simulink model "HeliDraft_25_03_2025"  (R2024b)
settings: Solver=VariableStepAuto  StartTime=0.0  StopTime=15  RelTol=1e-3
InitFcn:
  | if exist('MTOW', 'var') == 0
  |     set_param(gcs, 'SimulationCommand', 'stop');
  |     disp('HELICOPTER PARAMETERS ARE NOT DEFINED.');
  | end
values from neighbouring files (symbols this model uses):
  R = D/2    (= 2.01773704722)    [untitled.m]
undefined symbols (not defined in the file or in its folder): AngVel, AngVeltr, BatteryCap, BatteryDischrgRate, Coeffs, Earth, EngPowSL, hRef, Ion, Lfin, Lithium, MTOW, Preq2RPM, RPM2Vreq, VRef, WGS84
libraries: slpidlib x15, simulink x7, fl_lib x7, nesl_utility x6, simulink_extras x3, aerolibatmos2 x2, matrix_library x2, aerolibfltsims x2, aerolibtransform2 x1, shared6dof x1, aerolibconvert2 x1, batteryecm_lib x1
(part 1 of 3)
settings Model: Creator=stand-alone1  LastModifiedBy=stand-alone1

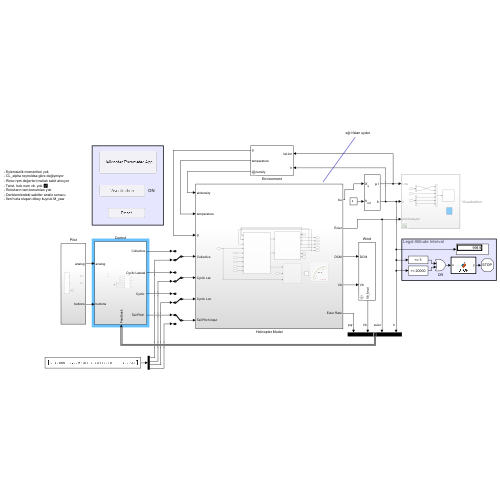
[thumbnail: Simulink's stored preview of the top-level diagram]
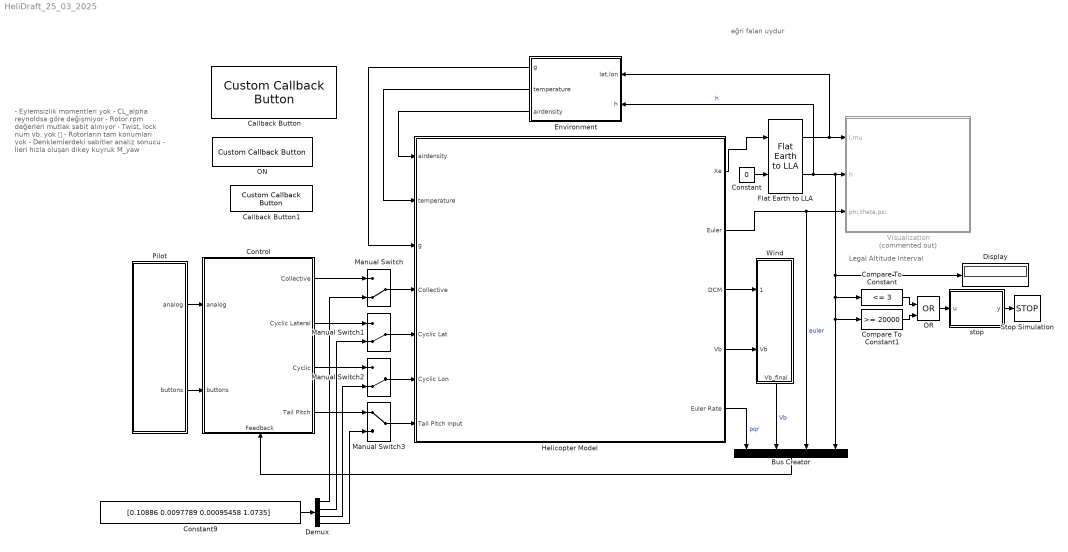
== system HeliDraft_25_03_2025 ==
  note: Legal Altitude Interval
  note: - Eylemsizlik momentleri yok
      | - CL_alpha reynoldsa göre değişmiyor
      | - Rotor rpm değerleri mutlak sabit alınıyor
      | - Twist, lock num vb. yok ✅
      | - Rotorların tam konumları yok
      | - Denklemlerdeki sabitler analiz sonucu
      | - İleri hızla oluşan dikey kuyruk M_yaw
  note: eğri falan uydur
  Bus Creator : BusCreator  Inputs=4
  Callback Button : CustomCallbackButton  Configuration="{\"components\":[{\"name\":\"BackgroundImageComponent\",\"settings\":{\"image\":{\"size\":[0,0],\"src\":\"default\",\"srcOrientation\":\"Right\"},\"position\":[0,0,1,1]}},{\"name\":\"ButtonStateComponent\",\"settings\":{\"buttonType\":\"momentary\",\"clickFcn\":\"run(\\\"HelicopterParameterEstimation.mlapp\\\");\",\"onValue\":1,\"position\":[0,0,1,1],\"pressDelay\":\"500\",\"pressFcn\":\"\",\"repeatInterval\":\"0\",\"states\":[{\"horizontalAlignment\":\"center\",\"image\":{\"position\":[0,0,1,1],\"size\":[1,1],\"src\":\"default\",\"srcOrientation\":\"Right\"},\"label\":{\"color\":[0.01176470588,0.01176470588,0.01176470588,1],\"icon\":{\"size\":[0,0],\"src\":\"default\",\"srcOrientation\":\"Right\"},\"iconOffset\":0,\"iconPlacement\":\"left\",\"opacity\":1,\"show\":true,\"text\":{\"content\":\"Helicopter Parameter App\",\"font\":\"Helvetica\"}},\"labelOffset\":[0,0],\"verticalAlignment\":\"middle\"},{\"horizontalAlignment\":\"center\",\"image\":{\"position\":[0,0,1,1],\"size\":[1,1],\"src\":\"default\",\"srcOrientation\":\"Right\"},\"label\":{\"color\":[0.01176470588,0.01176470588,0.01176470588,1],\"icon\":{\"size\":[0,0],\"src\":\"default\",\"srcOrientation\":\"Right\"},\"iconOffset\":0,\"iconPlacement\":\"left\",\"opacity\":1,\"show\":true,\"text\":{\"content\":\"Helicopter Parameter App\",\"font\":\"Helvetica\"}},\"labelOffset\":[0,0],\"verticalAlignment\":\"middle\"},{\"horizontalAlignment\":\"center\",\"image\":{\"position\":[0,0,1,1],\"size\":[1,1],\"src\":\"default\",\"srcOrientation\":\"Right\"},\"label\":{\"color\":[0.01176470588,0.01176470588,0.01176470588,1],\"icon\":{\"size\":[0,0],\"src\":\"default\",\"srcOrientation\":\"Right\"},\"iconOffset\":0,\"iconPlacement\":\"left\",\"opacity\":1,\"show\":true,\"text\":{\"content\":\"Helicopter Parameter App\",\"font\":\"Helvetica\"}},\"labelOffset\":[0,0],\"verticalAlignment\":\"middle\"},{\"horizontalAlignment\":\"center\",\"image\":{\"position\":[0,0,1,1],\"size\":[1,1],\"src\":\"default\",\"srcOrientation\":\"Right\"},\"label\":{\"color\":[0.01176470588,0.01176470588,0.01176470588,1],\"icon\":{\"size\":[0,0],\"src\":\"default\",\"srcOrientation\":\"Right\"},\"iconOffset\":0,\"iconPlacement\":\"left\",\"opacity\":1,\"show\":true,\"text\":{\"content\":\"Helicopter Parameter App\",\"font\":\"Helvetica\"}},\"labelOffset\":[0,0],\"verticalAlignment\":\"middle\"}]}},{\"name\":\"ForegroundImageComponent\",\"settings\":{\"image\":{\"size\":[0,0],\"src\":\"default\",\"srcOrientation\":\"Right\"},\"isForeground\":1,\"position\":[0,0,1,1]}}],\"settings\":{\"BindingType\":\"standalone\",\"backgroundColor\":[244,244,244,1],\"backgroundOffset\":0.2,\"backgroundOpacity\":1,\"fixedAspectRatio\":\"off\",\"foregroundColor\":[0.01176470588,0.01176470588,0.01176470588,1],\"migratedFromLegacy\":true,\"useBackgroundColor\":true,\"variant\":\"callback\",\"version\":\"R2023a\"},\"type\":\"Button\"}"  CustomBackgroundColor="{\"color\":[0.9568627451,0.9568627451,0.9568627451],\"show\":true}"
  Callback Button1 : CustomCallbackButton  Configuration="{\"components\":[{\"name\":\"BackgroundImageComponent\",\"settings\":{\"image\":{\"size\":[0,0],\"src\":\"default\",\"srcOrientation\":\"Right\"},\"position\":[0,0,1,1]}},{\"name\":\"ButtonStateComponent\",\"settings\":{\"buttonType\":\"momentary\",\"clickFcn\":\"clc; clear; close all;\",\"onValue\":1,\"position\":[0,0,1,1],\"pressDelay\":\"500\",\"pressFcn\":\"\",\"repeatInterval\":\"0\",\"states\":[{\"horizontalAlignment\":\"center\",\"image\":{\"position\":[0,0,1,1],\"size\":[1,1],\"src\":\"default\",\"srcOrientation\":\"Right\"},\"label\":{\"color\":[0.01176470588,0.01176470588,0.01176470588,1],\"icon\":{\"size\":[0,0],\"src\":\"default\",\"srcOrientation\":\"Right\"},\"iconOffset\":0,\"iconPlacement\":\"left\",\"opacity\":1,\"show\":true,\"text\":{\"content\":\"Reset\",\"font\":\"Helvetica\"}},\"labelOffset\":[0,0],\"verticalAlignment\":\"middle\"},{\"horizontalAlignment\":\"center\",\"image\":{\"position\":[0,0,1,1],\"size\":[1,1],\"src\":\"default\",\"srcOrientation\":\"Right\"},\"label\":{\"color\":[0.01176470588,0.01176470588,0.01176470588,1],\"icon\":{\"size\":[0,0],\"src\":\"default\",\"srcOrientation\":\"Right\"},\"iconOffset\":0,\"iconPlacement\":\"left\",\"opacity\":1,\"show\":true,\"text\":{\"content\":\"Reset\",\"font\":\"Helvetica\"}},\"labelOffset\":[0,0],\"verticalAlignment\":\"middle\"},{\"horizontalAlignment\":\"center\",\"image\":{\"position\":[0,0,1,1],\"size\":[1,1],\"src\":\"default\",\"srcOrientation\":\"Right\"},\"label\":{\"color\":[0.01176470588,0.01176470588,0.01176470588,1],\"icon\":{\"size\":[0,0],\"src\":\"default\",\"srcOrientation\":\"Right\"},\"iconOffset\":0,\"iconPlacement\":\"left\",\"opacity\":1,\"show\":true,\"text\":{\"content\":\"Reset\",\"font\":\"Helvetica\"}},\"labelOffset\":[0,0],\"verticalAlignment\":\"middle\"},{\"horizontalAlignment\":\"center\",\"image\":{\"position\":[0,0,1,1],\"size\":[1,1],\"src\":\"default\",\"srcOrientation\":\"Right\"},\"label\":{\"color\":[0.01176470588,0.01176470588,0.01176470588,1],\"icon\":{\"size\":[0,0],\"src\":\"default\",\"srcOrientation\":\"Right\"},\"iconOffset\":0,\"iconPlacement\":\"left\",\"opacity\":1,\"show\":true,\"text\":{\"content\":\"Reset\",\"font\":\"Helvetica\"}},\"labelOffset\":[0,0],\"verticalAlignment\":\"middle\"}]}},{\"name\":\"ForegroundImageComponent\",\"settings\":{\"image\":{\"size\":[0,0],\"src\":\"default\",\"srcOrientation\":\"Right\"},\"isForeground\":1,\"position\":[0,0,1,1]}}],\"settings\":{\"BindingType\":\"standalone\",\"backgroundColor\":[244,244,244,1],\"backgroundOffset\":0.2,\"backgroundOpacity\":1,\"fixedAspectRatio\":\"off\",\"foregroundColor\":[0.01176470588,0.01176470588,0.01176470588,1],\"migratedFromLegacy\":true,\"useBackgroundColor\":true,\"variant\":\"callback\",\"version\":\"R2023a\"},\"type\":\"Button\"}"  CustomBackgroundColor="{\"color\":[0.9568627451,0.9568627451,0.9568627451],\"show\":true}"
  Compare To Constant : simulink/Logic and Bit Operations/Compare To Constant  relop=<=  const=3  OutDataTypeStr=boolean
  Compare To Constant1 : simulink/Logic and Bit Operations/Compare To Constant  relop=>=  const=20000  OutDataTypeStr=boolean
  Constant : Constant  Value=0
  Constant9 : Constant  Value=[0.10886 0.0097789 0.00095458 1.0735]
  Control : Subsystem
      settings: PortSchema="{\"entries\":[{\"content\":{\"sides\":[{\"content\":{\"connectorIds\":[\"In1\",\"In2\"]},\"type\":\"ConnectorPlacement.EquallySpacedRectSide\",\"uuid\":\"00abb183-437f-4f12-ab32-5e5a492dbfa0\"},{\"content\":{\"connectorIds\":[\"Out1\",\"Out2\",\"Out3\",\"Out4\"],\"side\":\"RIGHT\"},\"type\":\"ConnectorPlacement.EquallySpacedRectSide\",\"uuid\":\"8c371a0c-8ad3-48b6-aeff-8a71ed38158f\"},{\"content\":{\"side\":\"TOP\"},\"type\":\"ConnectorPlacement.EquallySpacedRectSide\",\"uuid\":\"f88080f4-d031-401c-aadb-b0855552e319\"},{\"content\":{\"connectorIds\":[\"In3\"],\"side\":\"BOTTOM\"},\"type\":\"ConnectorPlacement.EquallySpacedRectSide\",\"uuid\":\"fa38cb5f-6d5a-488b-a33f-45554499d88c\"}]},\"type\":\"ConnectorPlacement.EquallySpacedConnector\",\"uuid\":\"58fada95-6377-4694-a368-953f0e4775f1\"}],\"packageUris\":[\"http://schema.mathworks.com/mf0/Connector/R2020b\"],\"version\":\"1.0\"}"
  Demux : Demux
  Display : Display
  Environment : Subsystem  mask{atmomodel=ISA, consg=on, Parameter3=on}
      mask prompts: atmomodel "Atmosphere Model"; consg "Constant g (Gravitational Acceleration)"; Parameter3 "On/Off"
      mask DialogControl a Prompt: Environment
      mask DialogControl b Prompt: Wind simulation, atmosphere properties and gravity model
      mask DialogControl Container4 Prompt: Environment
      mask DialogControl Container5 Prompt: Wind
  Flat Earth to LLA : aerolibtransform2/Flat Earth to LLA  units=Metric (MKS)  ptype=Earth (WGS84)  F=1/298.257223563  R=6378137  refPosPort=off  LL0=[0 10]  psi=0
  Helicopter Model : Subsystem
  Manual Switch : ManualSwitch  CurrentSetting=0
  Manual Switch1 : ManualSwitch  CurrentSetting=0
  Manual Switch2 : ManualSwitch  CurrentSetting=0
  Manual Switch3 : ManualSwitch
  ON : CustomCallbackButton  Configuration="{\"components\":[{\"name\":\"BackgroundImageComponent\",\"settings\":{\"image\":{\"size\":[0,0],\"src\":\"default\",\"srcOrientation\":\"Right\"},\"position\":[0,0,1,1]}},{\"name\":\"ButtonStateComponent\",\"settings\":{\"buttonType\":\"momentary\",\"clickFcn\":\"if strcmp(get_param('HeliDraft_05_03_2025\\/Visualization', 'Commented'), 'off')\\n    set_param('HeliDraft_05_03_2025\\/Visualization', 'Commented', 'on');\\n    set_param(\\\"HeliDraft_05_03_2025\\/ON\\\", 'Name', 'OFF');\\nelse\\n    set_param('HeliDraft_05_03_2025\\/Visualization', 'Commented', 'off');\\n    set_param(\\\"HeliDraft_05_03_2025\\/OFF\\\", 'Name', 'ON');\\nend\",\"onValue\":1,\"position\":[0,0,1,1],\"pressDelay\":\"500\",\"pressFcn\":\"\",\"repeatInterval\":\"0\",\"states\":[{\"horizontalAlignment\":\"center\",\"image\":{\"position\":[0,0,1,1],\"size\":[1,1],\"src\":\"default\",\"srcOrientation\":\"Right\"},\"label\":{\"color\":[0.01176470588,0.01176470588,0.01176470588,1],\"icon\":{\"size\":[0,0],\"src\":\"default\",\"srcOrientation\":\"Right\"},\"iconOffset\":0,\"iconPlacement\":\"left\",\"opacity\":1,\"show\":true,\"text\":{\"content\":\"Visualization\",\"font\":\"Helvetica\"}},\"labelOffset\":[0,0],\"verticalAlignment\":\"middle\"},{\"horizontalAlignment\":\"center\",\"image\":{\"position\":[0,0,1,1],\"size\":[1,1],\"src\":\"default\",\"srcOrientation\":\"Right\"},\"label\":{\"color\":[0.01176470588,0.01176470588,0.01176470588,1],\"icon\":{\"size\":[0,0],\"src\":\"default\",\"srcOrientation\":\"Right\"},\"iconOffset\":0,\"iconPlacement\":\"left\",\"opacity\":1,\"show\":true,\"text\":{\"content\":\"Visualization\",\"font\":\"Helvetica\"}},\"labelOffset\":[0,0],\"verticalAlignment\":\"middle\"},{\"horizontalAlignment\":\"center\",\"image\":{\"position\":[0,0,1,1],\"size\":[1,1],\"src\":\"default\",\"srcOrientation\":\"Right\"},\"label\":{\"color\":[0.01176470588,0.01176470588,0.01176470588,1],\"icon\":{\"size\":[0,0],\"src\":\"default\",\"srcOrientation\":\"Right\"},\"iconOffset\":0,\"iconPlacement\":\"left\",\"opacity\":1,\"show\":true,\"text\":{\"content\":\"Visualization\",\"font\":\"Helvetica\"}},\"labelOffset\":[0,0],\"verticalAlignment\":\"middle\"},{\"horizontalAlignment\":\"center\",\"image\":{\"position\":[0,0,1,1],\"size\":[1,1],\"src\":\"default\",\"srcOrientation\":\"Right\"},\"label\":{\"color\":[0.01176470588,0.01176470588,0.01176470588,1],\"icon\":{\"size\":[0,0],\"src\":\"default\",\"srcOrientation\":\"Right\"},\"iconOffset\":0,\"iconPlacement\":\"left\",\"opacity\":1,\"show\":true,\"text\":{\"content\":\"Visualization\",\"font\":\"Helvetica\"}},\"labelOffset\":[0,0],\"verticalAlignment\":\"middle\"}]}},{\"name\":\"ForegroundImageComponent\",\"settings\":{\"image\":{\"size\":[0,0],\"src\":\"default\",\"srcOrientation\":\"Right\"},\"isForeground\":1,\"position\":[0,0,1,1]}}],\"settings\":{\"BindingType\":\"standalone\",\"backgroundColor\":[244,244,244,1],\"backgroundOffset\":0.2,\"backgroundOpacity\":1,\"fixedAspectRatio\":\"off\",\"foregroundColor\":[0.01176470588,0.01176470588,0.01176470588,1],\"migratedFromLegacy\":true,\"useBackgroundColor\":true,\"variant\":\"callback\",\"version\":\"R2023a\"},\"type\":\"Button\"}"  CustomBackgroundColor="{\"color\":[0.9568627451,0.9568627451,0.9568627451],\"show\":true}"
  OR : Logic  Operator=OR  IconShape=distinctive  AllPortsSameDT=off  OutDataTypeStr=boolean
  Pilot : Subsystem
  Stop Simulation : Stop
  Visualization : Subsystem  Commented=on
  Wind : Subsystem  mask{windexist=on, wind2n=0, wind2e=0, wind2d=0, constwind=off, windstart=0, windend=0}
      mask prompts: windexist "On/Off"; wind2n "To North"; wind2e "To East"; wind2d "To Down"; constwind "Constant Wind"; windstart "Start"; windend "End"
      settings: PortSchema="{\"entries\":[{\"content\":{\"sides\":[{\"content\":{\"connectorIds\":[\"In1\",\"In2\"]},\"type\":\"ConnectorPlacement.EquallySpacedRectSide\",\"uuid\":\"c50a0b7f-10f6-4f94-9702-498138ee1021\"},{\"content\":{\"side\":\"RIGHT\"},\"type\":\"ConnectorPlacement.EquallySpacedRectSide\",\"uuid\":\"99b0af7a-d5f5-4d05-b84d-2e19e600cb93\"},{\"content\":{\"side\":\"TOP\"},\"type\":\"ConnectorPlacement.EquallySpacedRectSide\",\"uuid\":\"1ae8a906-0d49-4813-81f0-94e7246114b9\"},{\"content\":{\"connectorIds\":[\"Out1\"],\"side\":\"BOTTOM\"},\"type\":\"ConnectorPlacement.EquallySpacedRectSide\",\"uuid\":\"e4e64b9a-84af-456c-99c2-adf869c594cd\"}]},\"type\":\"ConnectorPlacement.EquallySpacedConnector\",\"uuid\":\"5fee7e0f-4ebe-498d-af71-6d032645fc1b\"}],\"packageUris\":[\"http://schema.mathworks.com/mf0/Connector/R2020b\"],\"version\":\"1.0\"}"
      mask DialogControl named Prompt: Wind Effect
      mask DialogControl Container2 Prompt: Time
  stop : MATLAB Function  TreatAsAtomicUnit=on
  wires:
  Constant/1 -> Flat Earth to LLA/2
  Flat Earth to LLA/1 -> Visualization/1(l,mu), Environment/1(lat,lon)
  Flat Earth to LLA/2 -> Display/1, Compare To Constant1/1, Bus Creator/4, Compare To Constant/1, Visualization/2(h), Environment/2(h)  "h"
  Pilot/1(analog) -> Control/1(analog)
  Pilot/2(buttons) -> Control/2(buttons)
  Environment/1(g) -> Helicopter Model/3(g)
  Environment/3(airdensity) -> Helicopter Model/1(airdensity)
  Helicopter Model/1(Xe) -> Flat Earth to LLA/1
  Helicopter Model/2(Euler) -> Visualization/3(phi,theta,psi), Bus Creator/3  "euler"
  Helicopter Model/4(Vb) -> Wind/2(Vb)
  Environment/2(temperature) -> Helicopter Model/2(temperature)
  Helicopter Model/5(Euler Rate) -> Bus Creator/1  "pqr"
  Control/1(Collective) -> Manual Switch/1
  Control/2(Cyclic Lateral) -> Manual Switch1/1
  Control/3("Cyclic ") -> Manual Switch2/1
  Control/4("Tail Pitch ") -> Manual Switch3/1
  Manual Switch/1 -> Helicopter Model/4(Collective)
  Manual Switch1/1 -> Helicopter Model/5(Cyclic Lat)
  Manual Switch2/1 -> Helicopter Model/6(Cyclic Lon)
  Manual Switch3/1 -> Helicopter Model/7(Tail Pitch input)
  OR/1 -> stop/1(u)
  Compare To Constant1/1 -> OR/2
  Compare To Constant/1 -> OR/1
  stop/1(y) -> Stop Simulation/1
  Helicopter Model/3(DCM) -> Wind/1(DCM)
  Wind/1(Vb_final) -> Bus Creator/2  "Vb"
  Demux/1 -> Manual Switch/2
  Demux/2 -> Manual Switch1/2
  Demux/3 -> Manual Switch2/2
  Demux/4 -> Manual Switch3/2
  Constant9/1 -> Demux/1
  Bus Creator/1 -> Control/3(Feedback)

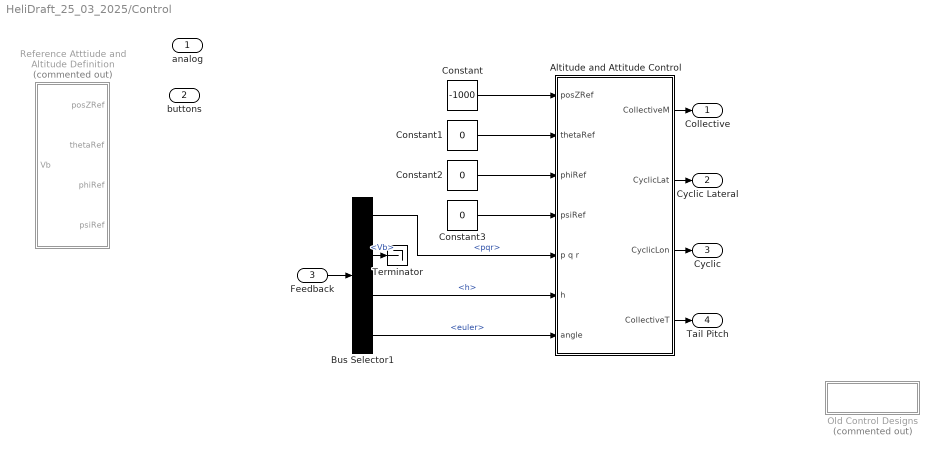
== system HeliDraft_25_03_2025/Control ==
  analog : Inport
  buttons : Inport  Port=2
  Feedback : Inport  Port=3
  Altitude and Attitude Control : Subsystem
  Bus Selector1 : BusSelector  OutputSignals=pqr,Vb,h,euler
  Constant : Constant  Value=-1000
  Constant1 : Constant  Value=0
  Constant2 : Constant  Value=0
  Constant3 : Constant  Value=0
  Old Control Designs : Subsystem  Commented=on
  Reference Atttiude and Altitude Definition : Subsystem  Commented=on
  Terminator : Terminator
  Collective : Outport
  Cyclic Lateral : Outport  Port=2
  "Cyclic " : Outport  Port=3
  "Tail Pitch " : Outport  Port=4
  wires:
  Altitude and Attitude Control/2(CyclicLat) -> Cyclic Lateral/1
  Altitude and Attitude Control/4(CollectiveT) -> "Tail Pitch "/1
  Altitude and Attitude Control/3(CyclicLon) -> "Cyclic "/1
  Constant3/1 -> Altitude and Attitude Control/4(psiRef)
  Constant2/1 -> Altitude and Attitude Control/3(phiRef)
  Altitude and Attitude Control/1(CollectiveM) -> Collective/1
  Constant1/1 -> Altitude and Attitude Control/2(thetaRef)
  Constant/1 -> Altitude and Attitude Control/1(posZRef)
  Feedback/1 -> Bus Selector1/1
  Bus Selector1/1 -> Altitude and Attitude Control/5(p q r)  "<pqr>"
  Bus Selector1/3 -> Altitude and Attitude Control/6(h)  "<h>"
  Bus Selector1/4 -> Altitude and Attitude Control/7(angle)  "<euler>"
  Bus Selector1/2 -> Terminator/1  "<Vb>"

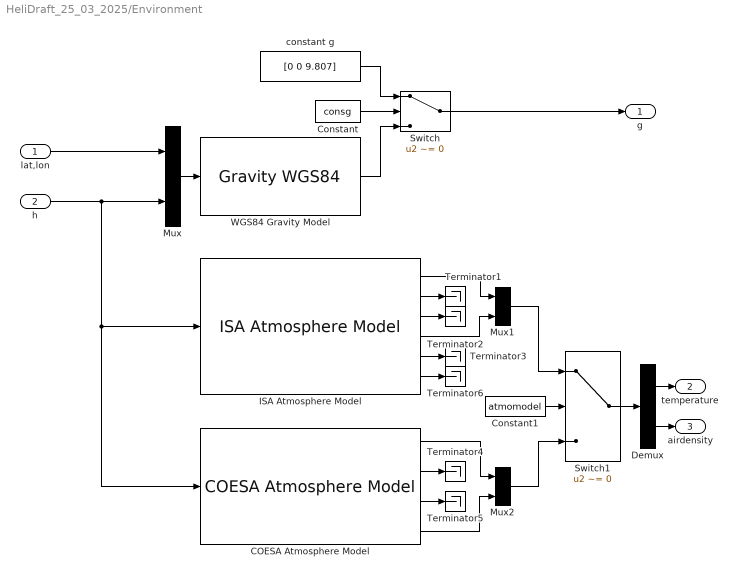
== system HeliDraft_25_03_2025/Environment ==
  lat,lon : Inport
  h : Inport  Port=2
  COESA Atmosphere Model : aerolibatmos2/COESA Atmosphere Model  units=Metric (MKS)  spec=1976 COESA-extended U.S. Standard Atmosphere  model=Profile  profile_var=High temperature  profile_percent=1%  profile_alt=5 km (16404 ft)  envelope_var=High temperature  envelope_percent=1%  action=Warning
  Constant : Constant  Value=consg
  Constant1 : Constant  Value=atmomodel
  Demux : Demux  Outputs=2
  ISA Atmosphere Model : aerolibatmos2/ISA Atmosphere Model  useExtended=off  action=Warning  custom=off  viscosityOut=on  g=9.80665  gamma=1.4  R=287.0531  L=0.0065  h_trop=11000  h_strat=20000  rho0=1.225  P0=101325  T0=288.15  h0=0  S=110.4  Tref=273.15  muref=1.716e-5
  Mux : Mux  Inputs=2
  Mux1 : Mux  Inputs=2
  Mux2 : Mux  Inputs=2
  Switch : Switch  Criteria=u2 ~= 0  SaturateOnIntegerOverflow=off  InputSameDT=off
  Switch1 : Switch  Criteria=u2 ~= 0  SaturateOnIntegerOverflow=off  InputSameDT=off
  Terminator{1..6} (6 alike) : Terminator
  "WGS84 Gravity Model  " : GravityWGS84
  constant g : Constant  Value=[0 0 9.807]
  g : Outport
  temperature : Outport  Port=2
  airdensity : Outport  Port=3
  wires:
  lat,lon/1 -> Mux/1
  Constant/1 -> Switch/2
  constant g/1 -> Switch/1
  "WGS84 Gravity Model  "/1 -> Switch/3
  Switch/1 -> g/1
  Mux/1 -> "WGS84 Gravity Model  "/1
  h/1 -> COESA Atmosphere Model/1, ISA Atmosphere Model/1, Mux/2
  Switch1/1 -> Demux/1
  ISA Atmosphere Model/1 -> Mux1/1
  ISA Atmosphere Model/2 -> Terminator1/1
  ISA Atmosphere Model/3 -> Terminator2/1
  COESA Atmosphere Model/2 -> Terminator4/1
  COESA Atmosphere Model/1 -> Mux2/1
  COESA Atmosphere Model/3 -> Terminator5/1
  ISA Atmosphere Model/4 -> Mux1/2
  COESA Atmosphere Model/4 -> Mux2/2
  Constant1/1 -> Switch1/2
  Mux1/1 -> Switch1/1
  Mux2/1 -> Switch1/3
  Demux/2 -> airdensity/1
  Demux/1 -> temperature/1
  ISA Atmosphere Model/5 -> Terminator3/1
  ISA Atmosphere Model/6 -> Terminator6/1

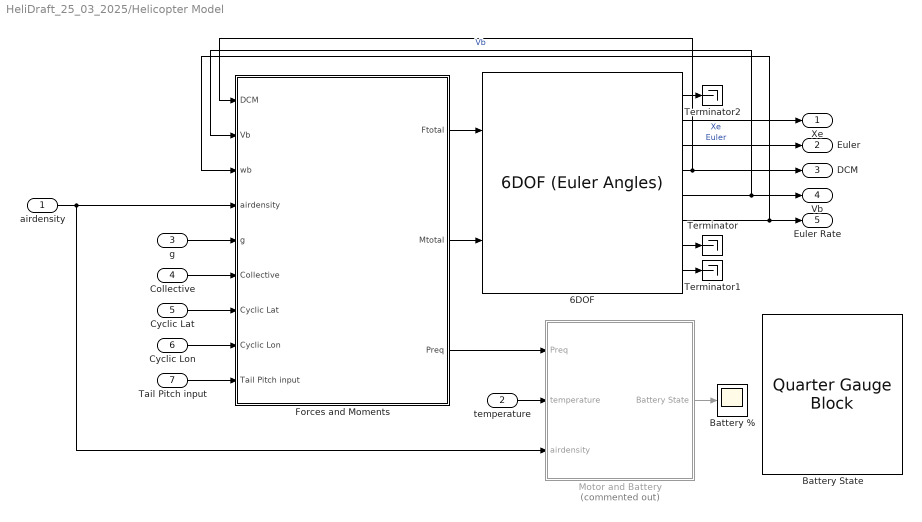
== system HeliDraft_25_03_2025/Helicopter Model ==
  airdensity : Inport
  temperature : Inport  Port=2
  g : Inport  Port=3
  Collective : Inport  Port=4
  Cyclic Lat : Inport  Port=5
  Cyclic Lon : Inport  Port=6
  Tail Pitch input : Inport  Port=7
  6DOF : shared6dof/6DOF (Euler Angles)  units=Metric (MKS)  mtype=Fixed  rep=Euler Angles  xme_0=[9.4779e-14 -1.5841e-13 -999.7936]  Vm_0=[3.4277e-06 0 0]  eul_0=[0.035989 -0.0070133 -4.6585e-14]  pm_0=[0 0 0]  mass_0=MTOW  mass_e=0.5  mass_f=2.0  inertia=[3795 0 2006;0 17259 0;0 0 14639]./100  inertia_e=eye(3)  inertia_f=2*eye(3)  k_quat=1.0  vre_flag=off  abi_flag=off  aMode=0  xme_statename=''  Vm_statename=''  eul_statename=''  quat_statename=''  pm_statename=''  mass_statename=''
  Battery % : Scope
  Battery State : QuarterGaugeBlock  LabelPosition=Hide
  Forces and Moments : Subsystem
  Motor and Battery : Subsystem  Commented=on
  Terminator : Terminator
  Terminator1 : Terminator
  Terminator2 : Terminator
  Xe : Outport
  Euler : Outport  Port=2
  DCM : Outport  Port=3
  Vb : Outport  Port=4
  Euler Rate : Outport  Port=5
  wires:
  6DOF/1 -> Terminator2/1
  6DOF/8 -> Terminator1/1
  Forces and Moments/1(Ftotal) -> 6DOF/1
  Forces and Moments/2(Mtotal) -> 6DOF/2
  6DOF/6 -> Forces and Moments/3(wb), Euler Rate/1
  6DOF/4 -> Forces and Moments/1(DCM), DCM/1
  6DOF/7 -> Terminator/1
  6DOF/5 -> Forces and Moments/2(Vb), Vb/1  "Vb"
  Cyclic Lat/1 -> Forces and Moments/7(Cyclic Lat)
  Collective/1 -> Forces and Moments/6(Collective)
  6DOF/3 -> Euler/1  "Euler"
  Tail Pitch input/1 -> Forces and Moments/9(Tail Pitch input)
  Cyclic Lon/1 -> Forces and Moments/8(Cyclic Lon)
  airdensity/1 -> Forces and Moments/4(airdensity), Motor and Battery/3(airdensity)
  g/1 -> Forces and Moments/5(g)
  6DOF/2 -> Xe/1  "Xe"
  Forces and Moments/3(Preq) -> Motor and Battery/1(Preq)
  Motor and Battery/1(Battery State) -> Battery %/1
  temperature/1 -> Motor and Battery/2(temperature)

== system HeliDraft_25_03_2025/Pilot ==
  Pilot Joystick All : aerolibanimutils/Pilot Joystick  JoystickID=None  OutputConfiguration=AllOutputs  SampleTime=1/30
      settings: LibrarySourceBlock=aerolibanimutils/Pilot Joystick All
  Terminator : Terminator
  analog : Outport
  buttons : Outport  Port=2
  wires:
  Pilot Joystick All/3 -> Terminator/1

== system HeliDraft_25_03_2025/Visualization ==
  l,mu : Inport
  h : Inport  Port=2
  phi,theta,psi : Inport  Port=3
  Demux : Demux  Outputs=2
  Demux1 : Demux  Outputs=3
  FlightGear Preconfigured 6DoF Animation : aerolibfltsims/FlightGear Preconfigured 6DoF Animation  xFlightGearVersion=v2019.1  DestinationIpAddress=127.0.0.1  DestinationPort=5502  SampleTime=1/30  packetVersion=24
  "Generate Run Script " : aerolibfltsims/Generate Run Script  Architecture=Default  dataFlow=Send  GeometryModelName=bo105  AirportId=KSFO  RunwayId=10L  InitialAltitude=7224  InitialHeading=113  OffsetDistance=4.72  OffsetAzimuth=0  InstallScenery=off  DisableShaders=on  OriginAddress=127.0.0.1  DestinationPort=5502  OriginPort=5505  LocalAddress=127.0.0.1  OutputFileName=runFlightGear.bat  FlightGearBaseDirectory=C:\Program Files\FlightGear 2020.3
  Mux : Mux  Inputs=6
  wires:
  l,mu/1 -> Demux/1
  Demux/2 -> Mux/1  "l"
  Demux/1 -> Mux/2  "mu"
  Mux/1 -> FlightGear Preconfigured 6DoF Animation/1
  h/1 -> Mux/3  "h"
  Demux1/1 -> Mux/4  "phi"
  Demux1/2 -> Mux/5  "theta"
  Demux1/3 -> Mux/6  "psi"
  phi,theta,psi/1 -> Demux1/1

== system HeliDraft_25_03_2025/Wind ==
  DCM : Inport
  Vb : Inport  Port=2
  AND : Logic  IconShape=distinctive  AllPortsSameDT=off  OutDataTypeStr=boolean
  AND_2 : Logic  IconShape=distinctive  AllPortsSameDT=off  OutDataTypeStr=boolean
  Add : Sum
  Clock : Clock
  Compare To Constant : simulink/Logic and Bit Operations/Compare To Constant  relop=>=  const=windstart  OutDataTypeStr=boolean
  Compare To Constant1 : simulink/Logic and Bit Operations/Compare To Constant  relop=<=  const=windend  OutDataTypeStr=boolean
  Constant : Constant  Value=windexist
  Constant1 : Constant  Value=constwind
  IsNonZero : simulink/Logic and Bit Operations/Compare To Zero  relop=~=  OutDataTypeStr=boolean
      settings: LibrarySourceBlock=|
      | simulink/Quick Insert/Logic and Bit
      | Operations/IsNonZero
  OR : Logic  Operator=OR  IconShape=distinctive  AllPortsSameDT=off  OutDataTypeStr=boolean
  Product : Product  Multiplication=Matrix(*)
  Switch : Switch  Criteria=u2 ~= 0  SaturateOnIntegerOverflow=off  InputSameDT=off
  Wind : Constant  Value=[wind2n wind2e wind2d]
  Vb_final : Outport
  wires:
  DCM/1 -> Product/1
  Add/1 -> Switch/1
  Vb/1 -> Switch/3, Add/2
  Wind/1 -> Product/2
  Product/1 -> Add/1
  Compare To Constant/1 -> AND/1
  Compare To Constant1/1 -> AND/2
  Clock/1 -> Compare To Constant/1, Compare To Constant1/1
  AND/1 -> OR/1
  Switch/1 -> Vb_final/1
  Constant/1 -> IsNonZero/1
  IsNonZero/1 -> AND_2/1
  AND_2/1 -> Switch/2
  OR/1 -> AND_2/2
  Constant1/1 -> OR/2

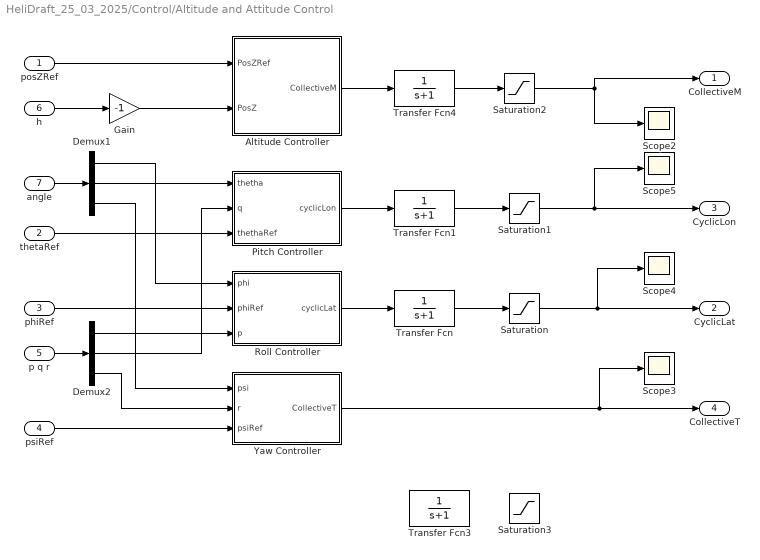
== system HeliDraft_25_03_2025/Control/Altitude and Attitude Control ==
  posZRef : Inport
  thetaRef : Inport  Port=2
  phiRef : Inport  Port=3
  psiRef : Inport  Port=4
  p q r : Inport  Port=5
  h : Inport  Port=6
  angle : Inport  Port=7
  Altitude Controller : Subsystem
  Demux1 : Demux  Outputs=3
  Demux2 : Demux  Outputs=3
  Gain : Gain  Gain=-1
  Pitch Controller : Subsystem
  Roll Controller : Subsystem
  Saturation : Saturate  UpperLimit=0.21  LowerLimit=-0.21
  Saturation1 : Saturate  UpperLimit=0.21  LowerLimit=-0.21
  Saturation2 : Saturate  UpperLimit=0.15  LowerLimit=0.08
  Saturation3 : Saturate  LowerLimit=0
  Scope{2..5} (4 alike) : Scope
  Transfer Fcn{,1,3..4} (4 alike) : TransferFcn  Denominator=[1 1]
  Yaw Controller : Subsystem
  CollectiveM : Outport
  CyclicLat : Outport  Port=2
  CyclicLon : Outport  Port=3
  CollectiveT : Outport  Port=4
  wires:
  psiRef/1 -> Yaw Controller/3(psiRef)
  h/1 -> Gain/1
  Demux2/1 -> Roll Controller/3(p)
  p q r/1 -> Demux2/1
  Saturation2/1 -> Scope2/1, CollectiveM/1
  Saturation/1 -> Scope4/1, CyclicLat/1
  Saturation1/1 -> CyclicLon/1, Scope5/1
  Transfer Fcn1/1 -> Saturation1/1
  Transfer Fcn/1 -> Saturation/1
  Roll Controller/1(cyclicLat) -> Transfer Fcn/1
  Demux2/2 -> Pitch Controller/2(q)
  Pitch Controller/1(cyclicLon) -> Transfer Fcn1/1
  angle/1 -> Demux1/1
  Demux1/1 -> Roll Controller/1(phi)
  Demux1/2 -> Pitch Controller/1(thetha)
  Transfer Fcn4/1 -> Saturation2/1
  Altitude Controller/1(CollectiveM) -> Transfer Fcn4/1
  Demux2/3 -> Yaw Controller/2(r)
  Demux1/3 -> Yaw Controller/1(psi)
  posZRef/1 -> Altitude Controller/1(PosZRef)
  thetaRef/1 -> Pitch Controller/3(thethaRef)
  phiRef/1 -> Roll Controller/2(phiRef)
  Gain/1 -> Altitude Controller/2(PosZ)
  Yaw Controller/1(CollectiveT) -> Scope3/1, CollectiveT/1

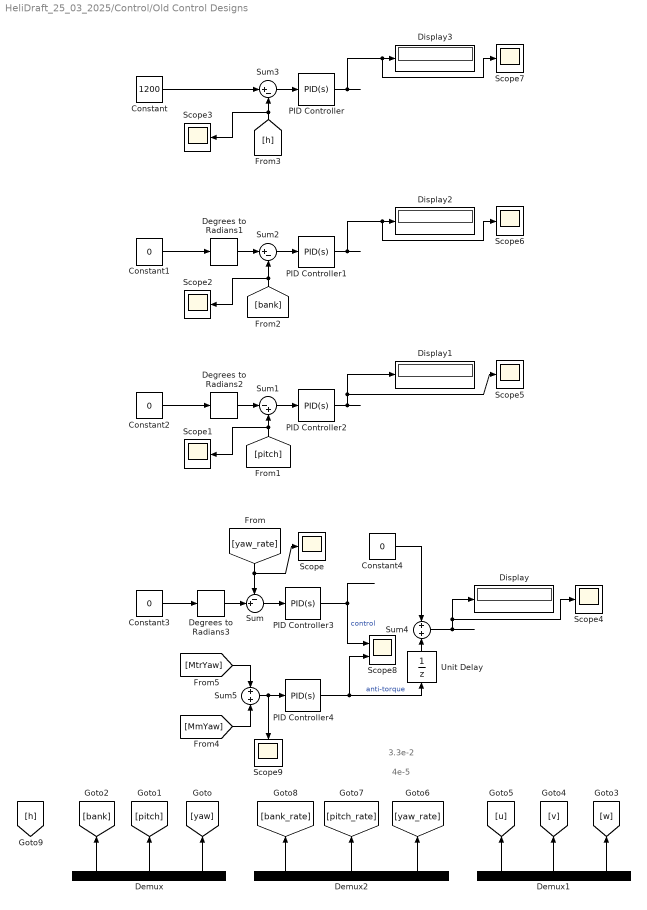
== system HeliDraft_25_03_2025/Control/Old Control Designs ==
  note: 3.3e-2
  note: 4e-5
  Constant : Constant  Value=1200
  Constant{1..4} (4 alike) : Constant  Value=0
  Degrees to Radians1 : simulink_extras/Transformations/Degrees to Radians
  Degrees to Radians2 : simulink_extras/Transformations/Degrees to Radians
  Degrees to Radians3 : simulink_extras/Transformations/Degrees to Radians
  Demux : Demux  Outputs=3
  Demux1 : Demux  Outputs=3
  Demux2 : Demux  Outputs=3
  Display{,1..3} (4 alike) : Display
      Display3 settings: Format=bank
  PID Controller : slpidlib/PID Controller  Controller=PID  Form=Parallel  TimeDomain=Continuous-time  UseExternalTs=off  SampleTime=-1  IntegratorMethod=Forward Euler  FilterMethod=Forward Euler  ControllerParametersSource=internal  P=1  I=1  UseKiTs=off  D=0  UseExternalDerivativeSource=off  N=100  UseFilter=on  TunerSelectOption=Transfer Function Based (PID Tuner App)  InitialConditionSource=internal  InitialConditionForIntegrator=0  InitialConditionForFilter=0  DifferentiatorICPrevScaledInput=0  ExternalReset=none  TrackingMode=off  Kt=1  LimitOutput=off  SatLimitsSource=internal  UpperSaturationLimit=inf  LowerSaturationLimit=-inf  LinearizeAsGain=on  AntiWindupMode=none  Kb=1  LimitIntegrator=off  UpperIntegratorSaturationLimit=inf  LowerIntegratorSaturationLimit=-inf  POutMin=[]  POutMax=[]  IOutMin=[]  IOutMax=[]  DOutMin=[]  DOutMax=[]  NOutMin=[]  NOutMax=[]  SumOutMin=[]  SumOutMax=[]  SaturationOutMin=[]  SaturationOutMax=[]  PParamMin=[]  PParamMax=[]  IParamMin=[]  IParamMax=[]  DParamMin=[]  DParamMax=[]  NParamMin=[]  NParamMax=[]  KbParamMin=[]  KbParamMax=[]  KtParamMin=[]  KtParamMax=[]  KbOutMin=[]  KbOutMax=[]  KtOutMin=[]  KtOutMax=[]  IntegratorOutMin=[]  IntegratorOutMax=[]  FilterOutMin=[]  FilterOutMax=[]  SumI1OutMin=[]  SumI1OutMax=[]  SumI2OutMin=[]  SumI2OutMax=[]  SumI3OutMin=[]  SumI3OutMax=[]  SumI4OutMin=[]  SumI4OutMax=[]  SumDOutMin=[]  SumDOutMax=[]  DifferentiatorOutMin=[]  DifferentiatorOutMax=[]  FilterDiffOutCoefMin=[]  FilterDiffOutCoefMax=[]  ReciprocalOutMin=[]  ReciprocalOutMax=[]  SumDenOutMin=[]  SumDenOutMax=[]  SumNumOutMin=[]  SumNumOutMax=[]  DivideOutMin=[]  DivideOutMax=[]  UdiffTsProdOutMin=[]  UdiffTsProdOutMax=[]  NTsProdOutMin=[]  NTsProdOutMax=[]  UintegralTsProdOutMin=[]  UintegralTsProdOutMax=[]  UngainTsProdOutMin=[]  UngainTsProdOutMax=[]  ClampingZeroOutDataTypeStr=Inherit: Inherit via back propagation  ClampingZeroOutMin=[]  ClampingZeroOutMax=[]  FilterDenConstantOutDataTypeStr=Inherit: Inherit via back propagation  FilterDenConstantOutMin=[]  FilterDenConstantOutMax=[]  PCopyOutDataTypeStr=Inherit: Inherit via back propagation  PCopyOutMin=[]  PCopyOutMax=[]  NCopyOutDataTypeStr=Inherit: Inherit via back propagation  NCopyOutMin=[]  NCopyOutMax=[]  IntegratorContinuousStateAttributes=''  IntegratorStateMustResolveToSignalObject=off  IntegratorRTWStateStorageClass=Auto  FilterContinuousStateAttributes=''  FilterStateMustResolveToSignalObject=off  FilterRTWStateStorageClass=Auto  ParallelPVariant=InternalParameters  IdealPVariant=Disabled  IVariant=InternalParameters  DVariant=InternalParameters  IntegratorVariant=Continuous  SatVariant=Disabled  AWVariant=Passthrough  PCopyVariant=Disabled  TRVariant=Disabled  FdbkBlocksVariant=Forward  IdealPFdbkVariant=Disabled  SatFdbkVariant=Disabled  DerivativeFilterVariant=ContFilter  NVariant=InternalParameters  NCopyVariant=Disabled  FilterICVariant=InternalICsFilter  IntegratorICVariant=InternalICs  ExternalResetVariant=Disabled  TRSumVariant=Passthrough  SumFdbkVariant=Disabled  SumVariant=Sum_PID  TsampFilterVariant=InternalTs  TsampNgainVariant=Passthrough  TsampIntegralVariant=Disabled_SignalSpec  ExternalSaturationOutDataTypeStr=Inherit: Same as second input  DerivativeSourceVariant=ErrorSignal  PreIntVariant=InternalPreInt
  PID Controller1 : slpidlib/PID Controller  Controller=PID  Form=Parallel  TimeDomain=Continuous-time  UseExternalTs=off  SampleTime=-1  IntegratorMethod=Forward Euler  FilterMethod=Forward Euler  ControllerParametersSource=internal  P=1  I=0  UseKiTs=off  D=0  UseExternalDerivativeSource=off  N=100  UseFilter=on  TunerSelectOption=Transfer Function Based (PID Tuner App)  InitialConditionSource=internal  InitialConditionForIntegrator=0  InitialConditionForFilter=0  DifferentiatorICPrevScaledInput=0  ExternalReset=none  TrackingMode=off  Kt=1  LimitOutput=off  SatLimitsSource=internal  UpperSaturationLimit=inf  LowerSaturationLimit=-inf  LinearizeAsGain=on  AntiWindupMode=none  Kb=1  LimitIntegrator=off  UpperIntegratorSaturationLimit=inf  LowerIntegratorSaturationLimit=-inf  POutMin=[]  POutMax=[]  IOutMin=[]  IOutMax=[]  DOutMin=[]  DOutMax=[]  NOutMin=[]  NOutMax=[]  SumOutMin=[]  SumOutMax=[]  SaturationOutMin=[]  SaturationOutMax=[]  PParamMin=[]  PParamMax=[]  IParamMin=[]  IParamMax=[]  DParamMin=[]  DParamMax=[]  NParamMin=[]  NParamMax=[]  KbParamMin=[]  KbParamMax=[]  KtParamMin=[]  KtParamMax=[]  KbOutMin=[]  KbOutMax=[]  KtOutMin=[]  KtOutMax=[]  IntegratorOutMin=[]  IntegratorOutMax=[]  FilterOutMin=[]  FilterOutMax=[]  SumI1OutMin=[]  SumI1OutMax=[]  SumI2OutMin=[]  SumI2OutMax=[]  SumI3OutMin=[]  SumI3OutMax=[]  SumI4OutMin=[]  SumI4OutMax=[]  SumDOutMin=[]  SumDOutMax=[]  DifferentiatorOutMin=[]  DifferentiatorOutMax=[]  FilterDiffOutCoefMin=[]  FilterDiffOutCoefMax=[]  ReciprocalOutMin=[]  ReciprocalOutMax=[]  SumDenOutMin=[]  SumDenOutMax=[]  SumNumOutMin=[]  SumNumOutMax=[]  DivideOutMin=[]  DivideOutMax=[]  UdiffTsProdOutMin=[]  UdiffTsProdOutMax=[]  NTsProdOutMin=[]  NTsProdOutMax=[]  UintegralTsProdOutMin=[]  UintegralTsProdOutMax=[]  UngainTsProdOutMin=[]  UngainTsProdOutMax=[]  ClampingZeroOutDataTypeStr=Inherit: Inherit via back propagation  ClampingZeroOutMin=[]  ClampingZeroOutMax=[]  FilterDenConstantOutDataTypeStr=Inherit: Inherit via back propagation  FilterDenConstantOutMin=[]  FilterDenConstantOutMax=[]  PCopyOutDataTypeStr=Inherit: Inherit via back propagation  PCopyOutMin=[]  PCopyOutMax=[]  NCopyOutDataTypeStr=Inherit: Inherit via back propagation  NCopyOutMin=[]  NCopyOutMax=[]  IntegratorContinuousStateAttributes=''  IntegratorStateMustResolveToSignalObject=off  IntegratorRTWStateStorageClass=Auto  FilterContinuousStateAttributes=''  FilterStateMustResolveToSignalObject=off  FilterRTWStateStorageClass=Auto  ParallelPVariant=InternalParameters  IdealPVariant=Disabled  IVariant=InternalParameters  DVariant=InternalParameters  IntegratorVariant=Continuous  SatVariant=Disabled  AWVariant=Passthrough  PCopyVariant=Disabled  TRVariant=Disabled  FdbkBlocksVariant=Forward  IdealPFdbkVariant=Disabled  SatFdbkVariant=Disabled  DerivativeFilterVariant=ContFilter  NVariant=InternalParameters  NCopyVariant=Disabled  FilterICVariant=InternalICsFilter  IntegratorICVariant=InternalICs  ExternalResetVariant=Disabled  TRSumVariant=Passthrough  SumFdbkVariant=Disabled  SumVariant=Sum_PID  TsampFilterVariant=InternalTs  TsampNgainVariant=Passthrough  TsampIntegralVariant=Disabled_SignalSpec  ExternalSaturationOutDataTypeStr=Inherit: Same as second input  DerivativeSourceVariant=ErrorSignal  PreIntVariant=InternalPreInt
  PID Controller2 : slpidlib/PID Controller  Controller=PID  Form=Parallel  TimeDomain=Continuous-time  UseExternalTs=off  SampleTime=-1  IntegratorMethod=Forward Euler  FilterMethod=Forward Euler  ControllerParametersSource=internal  P=30  I=0  UseKiTs=off  D=0  UseExternalDerivativeSource=off  N=100  UseFilter=on  TunerSelectOption=Transfer Function Based (PID Tuner App)  InitialConditionSource=internal  InitialConditionForIntegrator=0  InitialConditionForFilter=0  DifferentiatorICPrevScaledInput=0  ExternalReset=none  TrackingMode=off  Kt=1  LimitOutput=off  SatLimitsSource=internal  UpperSaturationLimit=inf  LowerSaturationLimit=-inf  LinearizeAsGain=on  AntiWindupMode=none  Kb=1  LimitIntegrator=off  UpperIntegratorSaturationLimit=inf  LowerIntegratorSaturationLimit=-inf  POutMin=[]  POutMax=[]  IOutMin=[]  IOutMax=[]  DOutMin=[]  DOutMax=[]  NOutMin=[]  NOutMax=[]  SumOutMin=[]  SumOutMax=[]  SaturationOutMin=[]  SaturationOutMax=[]  PParamMin=[]  PParamMax=[]  IParamMin=[]  IParamMax=[]  DParamMin=[]  DParamMax=[]  NParamMin=[]  NParamMax=[]  KbParamMin=[]  KbParamMax=[]  KtParamMin=[]  KtParamMax=[]  KbOutMin=[]  KbOutMax=[]  KtOutMin=[]  KtOutMax=[]  IntegratorOutMin=[]  IntegratorOutMax=[]  FilterOutMin=[]  FilterOutMax=[]  SumI1OutMin=[]  SumI1OutMax=[]  SumI2OutMin=[]  SumI2OutMax=[]  SumI3OutMin=[]  SumI3OutMax=[]  SumI4OutMin=[]  SumI4OutMax=[]  SumDOutMin=[]  SumDOutMax=[]  DifferentiatorOutMin=[]  DifferentiatorOutMax=[]  FilterDiffOutCoefMin=[]  FilterDiffOutCoefMax=[]  ReciprocalOutMin=[]  ReciprocalOutMax=[]  SumDenOutMin=[]  SumDenOutMax=[]  SumNumOutMin=[]  SumNumOutMax=[]  DivideOutMin=[]  DivideOutMax=[]  UdiffTsProdOutMin=[]  UdiffTsProdOutMax=[]  NTsProdOutMin=[]  NTsProdOutMax=[]  UintegralTsProdOutMin=[]  UintegralTsProdOutMax=[]  UngainTsProdOutMin=[]  UngainTsProdOutMax=[]  ClampingZeroOutDataTypeStr=Inherit: Inherit via back propagation  ClampingZeroOutMin=[]  ClampingZeroOutMax=[]  FilterDenConstantOutDataTypeStr=Inherit: Inherit via back propagation  FilterDenConstantOutMin=[]  FilterDenConstantOutMax=[]  PCopyOutDataTypeStr=Inherit: Inherit via back propagation  PCopyOutMin=[]  PCopyOutMax=[]  NCopyOutDataTypeStr=Inherit: Inherit via back propagation  NCopyOutMin=[]  NCopyOutMax=[]  IntegratorContinuousStateAttributes=''  IntegratorStateMustResolveToSignalObject=off  IntegratorRTWStateStorageClass=Auto  FilterContinuousStateAttributes=''  FilterStateMustResolveToSignalObject=off  FilterRTWStateStorageClass=Auto  ParallelPVariant=InternalParameters  IdealPVariant=Disabled  IVariant=InternalParameters  DVariant=InternalParameters  IntegratorVariant=Continuous  SatVariant=Disabled  AWVariant=Passthrough  PCopyVariant=Disabled  TRVariant=Disabled  FdbkBlocksVariant=Forward  IdealPFdbkVariant=Disabled  SatFdbkVariant=Disabled  DerivativeFilterVariant=ContFilter  NVariant=InternalParameters  NCopyVariant=Disabled  FilterICVariant=InternalICsFilter  IntegratorICVariant=InternalICs  ExternalResetVariant=Disabled  TRSumVariant=Passthrough  SumFdbkVariant=Disabled  SumVariant=Sum_PID  TsampFilterVariant=InternalTs  TsampNgainVariant=Passthrough  TsampIntegralVariant=Disabled_SignalSpec  ExternalSaturationOutDataTypeStr=Inherit: Same as second input  DerivativeSourceVariant=ErrorSignal  PreIntVariant=InternalPreInt
  PID Controller3 : slpidlib/PID Controller  Controller=PID  Form=Parallel  TimeDomain=Continuous-time  UseExternalTs=off  SampleTime=-1  IntegratorMethod=Forward Euler  FilterMethod=Forward Euler  ControllerParametersSource=internal  P=1e-6  I=0  UseKiTs=off  D=0  UseExternalDerivativeSource=off  N=100  UseFilter=on  TunerSelectOption=Transfer Function Based (PID Tuner App)  InitialConditionSource=internal  InitialConditionForIntegrator=0  InitialConditionForFilter=0  DifferentiatorICPrevScaledInput=0  ExternalReset=none  TrackingMode=off  Kt=1  LimitOutput=off  SatLimitsSource=internal  UpperSaturationLimit=inf  LowerSaturationLimit=-inf  LinearizeAsGain=on  AntiWindupMode=none  Kb=1  LimitIntegrator=off  UpperIntegratorSaturationLimit=inf  LowerIntegratorSaturationLimit=-inf  POutMin=[]  POutMax=[]  IOutMin=[]  IOutMax=[]  DOutMin=[]  DOutMax=[]  NOutMin=[]  NOutMax=[]  SumOutMin=[]  SumOutMax=[]  SaturationOutMin=[]  SaturationOutMax=[]  PParamMin=[]  PParamMax=[]  IParamMin=[]  IParamMax=[]  DParamMin=[]  DParamMax=[]  NParamMin=[]  NParamMax=[]  KbParamMin=[]  KbParamMax=[]  KtParamMin=[]  KtParamMax=[]  KbOutMin=[]  KbOutMax=[]  KtOutMin=[]  KtOutMax=[]  IntegratorOutMin=[]  IntegratorOutMax=[]  FilterOutMin=[]  FilterOutMax=[]  SumI1OutMin=[]  SumI1OutMax=[]  SumI2OutMin=[]  SumI2OutMax=[]  SumI3OutMin=[]  SumI3OutMax=[]  SumI4OutMin=[]  SumI4OutMax=[]  SumDOutMin=[]  SumDOutMax=[]  DifferentiatorOutMin=[]  DifferentiatorOutMax=[]  FilterDiffOutCoefMin=[]  FilterDiffOutCoefMax=[]  ReciprocalOutMin=[]  ReciprocalOutMax=[]  SumDenOutMin=[]  SumDenOutMax=[]  SumNumOutMin=[]  SumNumOutMax=[]  DivideOutMin=[]  DivideOutMax=[]  UdiffTsProdOutMin=[]  UdiffTsProdOutMax=[]  NTsProdOutMin=[]  NTsProdOutMax=[]  UintegralTsProdOutMin=[]  UintegralTsProdOutMax=[]  UngainTsProdOutMin=[]  UngainTsProdOutMax=[]  ClampingZeroOutDataTypeStr=Inherit: Inherit via back propagation  ClampingZeroOutMin=[]  ClampingZeroOutMax=[]  FilterDenConstantOutDataTypeStr=Inherit: Inherit via back propagation  FilterDenConstantOutMin=[]  FilterDenConstantOutMax=[]  PCopyOutDataTypeStr=Inherit: Inherit via back propagation  PCopyOutMin=[]  PCopyOutMax=[]  NCopyOutDataTypeStr=Inherit: Inherit via back propagation  NCopyOutMin=[]  NCopyOutMax=[]  IntegratorContinuousStateAttributes=''  IntegratorStateMustResolveToSignalObject=off  IntegratorRTWStateStorageClass=Auto  FilterContinuousStateAttributes=''  FilterStateMustResolveToSignalObject=off  FilterRTWStateStorageClass=Auto  ParallelPVariant=InternalParameters  IdealPVariant=Disabled  IVariant=InternalParameters  DVariant=InternalParameters  IntegratorVariant=Continuous  SatVariant=Disabled  AWVariant=Passthrough  PCopyVariant=Disabled  TRVariant=Disabled  FdbkBlocksVariant=Forward  IdealPFdbkVariant=Disabled  SatFdbkVariant=Disabled  DerivativeFilterVariant=ContFilter  NVariant=InternalParameters  NCopyVariant=Disabled  FilterICVariant=InternalICsFilter  IntegratorICVariant=InternalICs  ExternalResetVariant=Disabled  TRSumVariant=Passthrough  SumFdbkVariant=Disabled  SumVariant=Sum_PID  TsampFilterVariant=InternalTs  TsampNgainVariant=Passthrough  TsampIntegralVariant=Disabled_SignalSpec  ExternalSaturationOutDataTypeStr=Inherit: Same as second input  DerivativeSourceVariant=ErrorSignal  PreIntVariant=InternalPreInt
  PID Controller4 : slpidlib/PID Controller  Controller=PID  Form=Parallel  TimeDomain=Continuous-time  UseExternalTs=off  SampleTime=-1  IntegratorMethod=Forward Euler  FilterMethod=Forward Euler  ControllerParametersSource=internal  P=-5e-2  I=0  UseKiTs=off  D=0  UseExternalDerivativeSource=off  N=100  UseFilter=on  TunerSelectOption=Transfer Function Based (PID Tuner App)  InitialConditionSource=internal  InitialConditionForIntegrator=0  InitialConditionForFilter=0  DifferentiatorICPrevScaledInput=0  ExternalReset=none  TrackingMode=off  Kt=1  LimitOutput=off  SatLimitsSource=internal  UpperSaturationLimit=inf  LowerSaturationLimit=-inf  LinearizeAsGain=on  AntiWindupMode=none  Kb=1  LimitIntegrator=off  UpperIntegratorSaturationLimit=inf  LowerIntegratorSaturationLimit=-inf  POutMin=[]  POutMax=[]  IOutMin=[]  IOutMax=[]  DOutMin=[]  DOutMax=[]  NOutMin=[]  NOutMax=[]  SumOutMin=[]  SumOutMax=[]  SaturationOutMin=[]  SaturationOutMax=[]  PParamMin=[]  PParamMax=[]  IParamMin=[]  IParamMax=[]  DParamMin=[]  DParamMax=[]  NParamMin=[]  NParamMax=[]  KbParamMin=[]  KbParamMax=[]  KtParamMin=[]  KtParamMax=[]  KbOutMin=[]  KbOutMax=[]  KtOutMin=[]  KtOutMax=[]  IntegratorOutMin=[]  IntegratorOutMax=[]  FilterOutMin=[]  FilterOutMax=[]  SumI1OutMin=[]  SumI1OutMax=[]  SumI2OutMin=[]  SumI2OutMax=[]  SumI3OutMin=[]  SumI3OutMax=[]  SumI4OutMin=[]  SumI4OutMax=[]  SumDOutMin=[]  SumDOutMax=[]  DifferentiatorOutMin=[]  DifferentiatorOutMax=[]  FilterDiffOutCoefMin=[]  FilterDiffOutCoefMax=[]  ReciprocalOutMin=[]  ReciprocalOutMax=[]  SumDenOutMin=[]  SumDenOutMax=[]  SumNumOutMin=[]  SumNumOutMax=[]  DivideOutMin=[]  DivideOutMax=[]  UdiffTsProdOutMin=[]  UdiffTsProdOutMax=[]  NTsProdOutMin=[]  NTsProdOutMax=[]  UintegralTsProdOutMin=[]  UintegralTsProdOutMax=[]  UngainTsProdOutMin=[]  UngainTsProdOutMax=[]  ClampingZeroOutDataTypeStr=Inherit: Inherit via back propagation  ClampingZeroOutMin=[]  ClampingZeroOutMax=[]  FilterDenConstantOutDataTypeStr=Inherit: Inherit via back propagation  FilterDenConstantOutMin=[]  FilterDenConstantOutMax=[]  PCopyOutDataTypeStr=Inherit: Inherit via back propagation  PCopyOutMin=[]  PCopyOutMax=[]  NCopyOutDataTypeStr=Inherit: Inherit via back propagation  NCopyOutMin=[]  NCopyOutMax=[]  IntegratorContinuousStateAttributes=''  IntegratorStateMustResolveToSignalObject=off  IntegratorRTWStateStorageClass=Auto  FilterContinuousStateAttributes=''  FilterStateMustResolveToSignalObject=off  FilterRTWStateStorageClass=Auto  ParallelPVariant=InternalParameters  IdealPVariant=Disabled  IVariant=InternalParameters  DVariant=InternalParameters  IntegratorVariant=Continuous  SatVariant=Disabled  AWVariant=Passthrough  PCopyVariant=Disabled  TRVariant=Disabled  FdbkBlocksVariant=Forward  IdealPFdbkVariant=Disabled  SatFdbkVariant=Disabled  DerivativeFilterVariant=ContFilter  NVariant=InternalParameters  NCopyVariant=Disabled  FilterICVariant=InternalICsFilter  IntegratorICVariant=InternalICs  ExternalResetVariant=Disabled  TRSumVariant=Passthrough  SumFdbkVariant=Disabled  SumVariant=Sum_PID  TsampFilterVariant=InternalTs  TsampNgainVariant=Passthrough  TsampIntegralVariant=Disabled_SignalSpec  ExternalSaturationOutDataTypeStr=Inherit: Same as second input  DerivativeSourceVariant=ErrorSignal  PreIntVariant=InternalPreInt
  Scope{,1..7,9} (9 alike) : Scope
  Scope8 : Scope  NumInputPorts=2
  Sum : Sum  Inputs=-+|
  Sum1 : Sum  Inputs=|-+
  Sum2 : Sum  Inputs=|+-
  Sum3 : Sum  Inputs=|+-
  Sum4 : Sum  Inputs=+|+
  Sum5 : Sum  Inputs=+|+
  Unit Delay : UnitDelay  InitialCondition=6.6051081  SampleTime=-1  HasFrameUpgradeWarning=on
  wires:
  Constant3/1 -> Degrees to Radians3/1
  ? -> Demux1/1
  Demux/2 -> [pitch]
  ? -> [h]
  Sum/1 -> PID Controller3/1
  Demux1/2 -> [v]
  PID Controller2/1 -> Display1/1, Scope5/1
  Demux/3 -> [yaw]
  Unit Delay/1 -> Sum4/2
  Constant2/1 -> Degrees to Radians2/1
  Constant1/1 -> Degrees to Radians1/1
  Sum2/1 -> PID Controller1/1
  Constant4/1 -> Sum4/1
  [pitch] -> Scope1/1, Sum1/2
  PID Controller4/1 -> Unit Delay/1, Scope8/2  "anti-torque"
  [MmYaw] -> Sum5/2
  Constant/1 -> Sum3/1
  ? -> Demux2/1
  Degrees to Radians2/1 -> Sum1/1
  Sum5/1 -> PID Controller4/1, Scope9/1
  Demux1/3 -> [w]
  [bank] -> Scope2/1, Sum2/2
  Demux1/1 -> [u]
  PID Controller/1 -> Scope7/1, Display3/1
  [yaw_rate] -> Scope/1, Sum/1
  [MtrYaw] -> Sum5/1
  Demux2/1 -> [bank_rate]
  Degrees to Radians1/1 -> Sum2/1
  Demux2/2 -> [pitch_rate]
  Demux/1 -> [bank]
  Degrees to Radians3/1 -> Sum/2
  PID Controller3/1 -> Scope8/1  "control"
  Demux2/3 -> [yaw_rate]
  ? -> Demux/1
  Sum4/1 -> Display/1, Scope4/1
  [h] -> Scope3/1, Sum3/2
  Sum1/1 -> PID Controller2/1
  Sum3/1 -> PID Controller/1
  PID Controller1/1 -> Scope6/1, Display2/1

== system HeliDraft_25_03_2025/Control/Reference Atttiude and Altitude Definition ==
  Vb : Inport
  Constant1 : Constant  Value=0
  Constant2 : Constant  Value=0
  Demux3 : Demux  Outputs=3
  Forward Velocity Control : Subsystem
  Lateral Velocity Control : Subsystem
  Ramp : simulink/Sources/Ramp  slope=8  start=0  InitialOutput=0
  Saturation : Saturate  UpperLimit=hRef  LowerLimit=0
  Terminator : Terminator
  Variant Subsystem : Subsystem  Variant=on
  posZRef : Outport
  thetaRef : Outport  Port=2
  phiRef : Outport  Port=3
  psiRef : Outport  Port=4
  wires:
  Constant1/1 -> Lateral Velocity Control/1(speedvRef)
  Vb/1 -> Variant Subsystem/1(Vb), Demux3/1
  Lateral Velocity Control/1(phiRef) -> phiRef/1
  Forward Velocity Control/1(thetaRef) -> thetaRef/1
  Constant2/1 -> psiRef/1
  Ramp/1 -> Saturation/1
  Saturation/1 -> posZRef/1
  Demux3/3 -> Terminator/1
  Variant Subsystem/1(ub) -> Forward Velocity Control/1(speeduRef)
  Demux3/1 -> Forward Velocity Control/2(ub)
  Demux3/2 -> Lateral Velocity Control/2(vb)

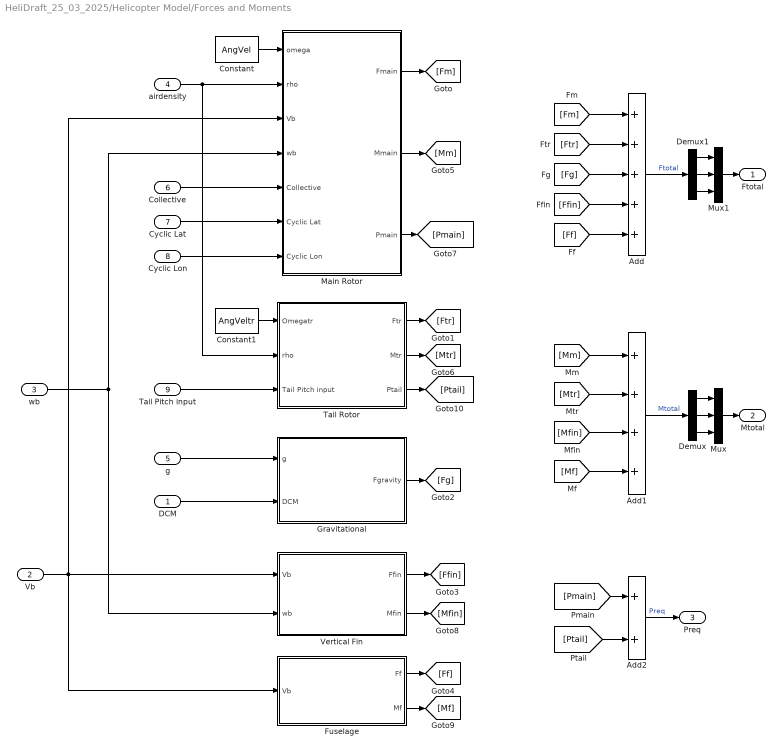
== system HeliDraft_25_03_2025/Helicopter Model/Forces and Moments ==
  DCM : Inport
  Vb : Inport  Port=2
  wb : Inport  Port=3
  airdensity : Inport  Port=4
  g : Inport  Port=5
  Collective : Inport  Port=6
  Cyclic Lat : Inport  Port=7
  Cyclic Lon : Inport  Port=8
  Tail Pitch input : Inport  Port=9
  Add : Sum  Inputs=+++++
  Add1 : Sum  Inputs=++++
  Add2 : Sum
  Constant : Constant  Value=AngVel
  Constant1 : Constant  Value=AngVeltr
  Demux : Demux  Outputs=3
  Demux1 : Demux  Outputs=3
  Fuselage : Subsystem
  Gravitational : Subsystem
  Main Rotor : Subsystem
  Mux : Mux  Inputs=3
  Mux1 : Mux  Inputs=3
  Tail Rotor : Subsystem
  Vertical Fin : Subsystem
  Ftotal : Outport
  Mtotal : Outport  Port=2
  Preq : Outport  Port=3
  wires:
  Add/1 -> Demux1/1  "Ftotal"
  Add1/1 -> Demux/1  "Mtotal"
  Main Rotor/1(Fmain) -> [Fm]
  Tail Rotor/1(Ftr) -> [Ftr]
  Gravitational/1(Fgravity) -> [Fg]
  Vertical Fin/1(Ffin) -> [Ffin]
  [Fm] -> Add/1
  [Ftr] -> Add/2
  [Fg] -> Add/3
  [Ffin] -> Add/4
  [Ff] -> Add/5
  Main Rotor/2(Mmain) -> [Mm]
  Tail Rotor/2(Mtr) -> [Mtr]
  Vertical Fin/2(Mfin) -> [Mfin]
  [Mm] -> Add1/1
  [Mtr] -> Add1/2
  [Mf] -> Add1/4
  [Mfin] -> Add1/3
  Constant/1 -> Main Rotor/1(omega)
  Constant1/1 -> Tail Rotor/1(Omegatr)
  airdensity/1 -> Tail Rotor/2(rho), Main Rotor/2(rho)
  g/1 -> Gravitational/1(g)
  DCM/1 -> Gravitational/2(DCM)
  Collective/1 -> Main Rotor/5(Collective)
  Tail Pitch input/1 -> Tail Rotor/3(Tail Pitch input)
  Cyclic Lat/1 -> Main Rotor/6(Cyclic Lat)
  Cyclic Lon/1 -> Main Rotor/7(Cyclic Lon)
  wb/1 -> Main Rotor/4(wb), Vertical Fin/2(wb)
  Vb/1 -> Fuselage/1(Vb), Main Rotor/3(Vb), Vertical Fin/1(Vb)
  Add2/1 -> Preq/1  "Preq"
  Main Rotor/3(Pmain) -> [Pmain]
  Tail Rotor/3(Ptail) -> [Ptail]
  [Pmain] -> Add2/1
  [Ptail] -> Add2/2
  Fuselage/1(Ff) -> [Ff]
  Fuselage/2(Mf) -> [Mf]
  Mux/1 -> Mtotal/1
  Demux/3 -> Mux/3
  Demux/2 -> Mux/2
  Demux1/2 -> Mux1/2
  Demux1/3 -> Mux1/3
  Mux1/1 -> Ftotal/1
  Demux/1 -> Mux/1
  Demux1/1 -> Mux1/1
